simulink model "Simulink_Program"  (R2023b)
settings: Solver=VariableStepAuto  StartTime=0.0  StopTime=1  RelTol=1e-3
undefined symbols (not defined in the file): battery_builder_rtmsupport, gcbh, Ns_Module, NumModules
libraries: nesl_utility x52, BatteryPack_105s34p_Library_lib x36, fl_lib x17, ee_lib x7
(part 2 of 5)

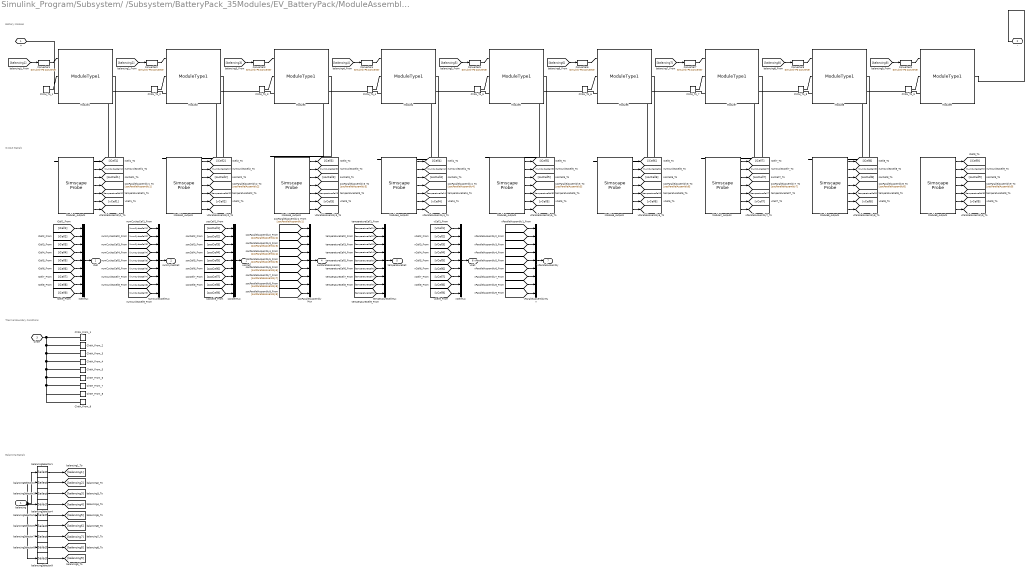
== system Simulink_Program/Subsystem/ /Subsystem/BatteryPack_35Modules/EV_BatteryPack/ModuleAssembly1 ==
  note: Balancing Signals
  note: Thermal Boundary Conditions
  note: Output Signals
  note: Battery Modules
  balancing : Inport  PortDimensions=27
  ClntH_From_1 : ConnectionLabel  Label=clntH_1
  ClntH_From_2 : ConnectionLabel  Label=clntH_2
  ClntH_From_3 : ConnectionLabel  Label=clntH_3
  ClntH_From_4 : ConnectionLabel  Label=clntH_4
  ClntH_From_5 : ConnectionLabel  Label=clntH_5
  ClntH_From_6 : ConnectionLabel  Label=clntH_6
  ClntH_From_7 : ConnectionLabel  Label=clntH_7
  ClntH_From_8 : ConnectionLabel  Label=clntH_8
  ClntH_From_9 : ConnectionLabel  Label=clntH_9
  ClntH_To_1 : ConnectionLabel  Label=clntH_1
  ClntH_To_2 : ConnectionLabel  Label=clntH_2
  ClntH_To_3 : ConnectionLabel  Label=clntH_3
  ClntH_To_4 : ConnectionLabel  Label=clntH_4
  ClntH_To_5 : ConnectionLabel  Label=clntH_5
  ClntH_To_6 : ConnectionLabel  Label=clntH_6
  ClntH_To_7 : ConnectionLabel  Label=clntH_7
  ClntH_To_8 : ConnectionLabel  Label=clntH_8
  ClntH_To_9 : ConnectionLabel  Label=clntH_9
  Converter{1..9} (9 alike) : nesl_utility/Simulink-PS Converter  PhysicalDomain=network_engine_domain  SubClassName=ps_input  LeftPortType=input  RightPortType=output  PseudoPeriodic=off  Frequencies=[]  NoiseDistribution=none  NoiseParameters=[]  Unit=1  AffineConversion=off  FilteringAndDerivatives=provide  SimscapeFilterOrder=1  InputFilterTimeConstant=0.001  UdotUserProvided=0
  Module1 : BatteryPack_105s34p_Library_lib/Modules/ModuleType1  SOC_vecCell=ModuleType1.SOC_vecCell  T_vecCell=ModuleType1.T_vecCell K  V0_matCell=ModuleType1.V0_matCell V  V_rangeCell=ModuleType1.V_rangeCell V  R0_matCell=ModuleType1.R0_matCell Ohm  AHCell=ModuleType1.AHCell A*hr  extrapolation_optionCell=simscape.enum.extrapolation.nearest  thermal_massCell=ModuleType1.thermal_massCell J/K  CoolantResistance=ModuleType1.CoolantResistance K/W  CellBalancingClosedResistance=ModuleType1.CellBalancingClosedResistance Ohm  CellBalancingOpenConductance=ModuleType1.CellBalancingOpenConductance 1/Ohm  CellBalancingThreshold=ModuleType1.CellBalancingThreshold  CellBalancingResistance=ModuleType1.CellBalancingResistance Ohm  P=34  S=3  iCell_specify=on  iCell_priority=None  iCell=ModuleAssembly1.Module1.iCell A  iCell_nominal_specify=off  iCell_nominal_unit=A  iCell_nominal_value=1  vCell_specify=on  vCell_priority=None  vCell=ModuleAssembly1.Module1.vCell V  vCell_nominal_specify=off  vCell_nominal_unit=V  vCell_nominal_value=1  socCell_specify=on  socCell_priority=High  socCell=ModuleAssembly1.Module1.socCell  socCell_nominal_specify=off  socCell_nominal_unit=1  socCell_nominal_value=1  numCyclesCell_specify=on  numCyclesCell_priority=High  numCyclesCell=ModuleAssembly1.Module1.numCyclesCell  numCyclesCell_nominal_specify=off  numCyclesCell_nominal_unit=1  numCyclesCell_nominal_value=1  temperatureCell_specify=on  temperatureCell_priority=High  temperatureCell=ModuleAssembly1.Module1.temperatureCell K  temperatureCell_nominal_specify=off  temperatureCell_nominal_unit=K  temperatureCell_nominal_value=1  vParallelAssembly_specify=on  vParallelAssembly_priority=None  vParallelAssembly=ModuleAssembly1.Module1.vParallelAssembly V  vParallelAssembly_nominal_specify=off  vParallelAssembly_nominal_unit=V  vParallelAssembly_nominal_value=1  socParallelAssembly_specify=on  socParallelAssembly_priority=None  socParallelAssembly=ModuleAssembly1.Module1.socParallelAssembly  socParallelAssembly_nominal_specify=off  socParallelAssembly_nominal_unit=1  socParallelAssembly_nominal_value=1
      settings: InternalSimscapePortConfiguration="{\"Bottom\":[{\"id\":\"n\",\"label\":\"-\",\"type\":\"foundation.electrical.electrical\"}],\"Left\":[{\"id\":\"enableCellBalancing\",\"label\":\"CB\",\"type\":\"input\"},{\"id\":\"ClntH\",\"label\":\"ClntH\",\"type\":\"foundation.thermal.thermal\"}],\"Right\":[],\"Top\":[{\"id\":\"p\",\"label\":\"+\",\"type\":\"foundation.electrical.electrical\"}]}"
  Module1_outputs : SimscapeProbe  BoundBlock=363  Variables={iCell, numCyclesCell, socCell, socParallelAssembly, temperatureCell, vCell, vParallelAssembly}
  Module2 : BatteryPack_105s34p_Library_lib/Modules/ModuleType1  SOC_vecCell=ModuleType1.SOC_vecCell  T_vecCell=ModuleType1.T_vecCell K  V0_matCell=ModuleType1.V0_matCell V  V_rangeCell=ModuleType1.V_rangeCell V  R0_matCell=ModuleType1.R0_matCell Ohm  AHCell=ModuleType1.AHCell A*hr  extrapolation_optionCell=simscape.enum.extrapolation.nearest  thermal_massCell=ModuleType1.thermal_massCell J/K  CoolantResistance=ModuleType1.CoolantResistance K/W  CellBalancingClosedResistance=ModuleType1.CellBalancingClosedResistance Ohm  CellBalancingOpenConductance=ModuleType1.CellBalancingOpenConductance 1/Ohm  CellBalancingThreshold=ModuleType1.CellBalancingThreshold  CellBalancingResistance=ModuleType1.CellBalancingResistance Ohm  P=34  S=3  iCell_specify=on  iCell_priority=None  iCell=ModuleAssembly1.Module2.iCell A  iCell_nominal_specify=off  iCell_nominal_unit=A  iCell_nominal_value=1  vCell_specify=on  vCell_priority=None  vCell=ModuleAssembly1.Module2.vCell V  vCell_nominal_specify=off  vCell_nominal_unit=V  vCell_nominal_value=1  socCell_specify=on  socCell_priority=High  socCell=ModuleAssembly1.Module2.socCell  socCell_nominal_specify=off  socCell_nominal_unit=1  socCell_nominal_value=1  numCyclesCell_specify=on  numCyclesCell_priority=High  numCyclesCell=ModuleAssembly1.Module2.numCyclesCell  numCyclesCell_nominal_specify=off  numCyclesCell_nominal_unit=1  numCyclesCell_nominal_value=1  temperatureCell_specify=on  temperatureCell_priority=High  temperatureCell=ModuleAssembly1.Module2.temperatureCell K  temperatureCell_nominal_specify=off  temperatureCell_nominal_unit=K  temperatureCell_nominal_value=1  vParallelAssembly_specify=on  vParallelAssembly_priority=None  vParallelAssembly=ModuleAssembly1.Module2.vParallelAssembly V  vParallelAssembly_nominal_specify=off  vParallelAssembly_nominal_unit=V  vParallelAssembly_nominal_value=1  socParallelAssembly_specify=on  socParallelAssembly_priority=None  socParallelAssembly=ModuleAssembly1.Module2.socParallelAssembly  socParallelAssembly_nominal_specify=off  socParallelAssembly_nominal_unit=1  socParallelAssembly_nominal_value=1
      settings: InternalSimscapePortConfiguration="{\"Bottom\":[{\"id\":\"n\",\"label\":\"-\",\"type\":\"foundation.electrical.electrical\"}],\"Left\":[{\"id\":\"enableCellBalancing\",\"label\":\"CB\",\"type\":\"input\"},{\"id\":\"ClntH\",\"label\":\"ClntH\",\"type\":\"foundation.thermal.thermal\"}],\"Right\":[],\"Top\":[{\"id\":\"p\",\"label\":\"+\",\"type\":\"foundation.electrical.electrical\"}]}"
  Module2_outputs : SimscapeProbe  BoundBlock=365  Variables={iCell, numCyclesCell, socCell, socParallelAssembly, temperatureCell, vCell, vParallelAssembly}
  Module3 : BatteryPack_105s34p_Library_lib/Modules/ModuleType1  SOC_vecCell=ModuleType1.SOC_vecCell  T_vecCell=ModuleType1.T_vecCell K  V0_matCell=ModuleType1.V0_matCell V  V_rangeCell=ModuleType1.V_rangeCell V  R0_matCell=ModuleType1.R0_matCell Ohm  AHCell=ModuleType1.AHCell A*hr  extrapolation_optionCell=simscape.enum.extrapolation.nearest  thermal_massCell=ModuleType1.thermal_massCell J/K  CoolantResistance=ModuleType1.CoolantResistance K/W  CellBalancingClosedResistance=ModuleType1.CellBalancingClosedResistance Ohm  CellBalancingOpenConductance=ModuleType1.CellBalancingOpenConductance 1/Ohm  CellBalancingThreshold=ModuleType1.CellBalancingThreshold  CellBalancingResistance=ModuleType1.CellBalancingResistance Ohm  P=34  S=3  iCell_specify=on  iCell_priority=None  iCell=ModuleAssembly1.Module3.iCell A  iCell_nominal_specify=off  iCell_nominal_unit=A  iCell_nominal_value=1  vCell_specify=on  vCell_priority=None  vCell=ModuleAssembly1.Module3.vCell V  vCell_nominal_specify=off  vCell_nominal_unit=V  vCell_nominal_value=1  socCell_specify=on  socCell_priority=High  socCell=ModuleAssembly1.Module3.socCell  socCell_nominal_specify=off  socCell_nominal_unit=1  socCell_nominal_value=1  numCyclesCell_specify=on  numCyclesCell_priority=High  numCyclesCell=ModuleAssembly1.Module3.numCyclesCell  numCyclesCell_nominal_specify=off  numCyclesCell_nominal_unit=1  numCyclesCell_nominal_value=1  temperatureCell_specify=on  temperatureCell_priority=High  temperatureCell=ModuleAssembly1.Module3.temperatureCell K  temperatureCell_nominal_specify=off  temperatureCell_nominal_unit=K  temperatureCell_nominal_value=1  vParallelAssembly_specify=on  vParallelAssembly_priority=None  vParallelAssembly=ModuleAssembly1.Module3.vParallelAssembly V  vParallelAssembly_nominal_specify=off  vParallelAssembly_nominal_unit=V  vParallelAssembly_nominal_value=1  socParallelAssembly_specify=on  socParallelAssembly_priority=None  socParallelAssembly=ModuleAssembly1.Module3.socParallelAssembly  socParallelAssembly_nominal_specify=off  socParallelAssembly_nominal_unit=1  socParallelAssembly_nominal_value=1
      settings: InternalSimscapePortConfiguration="{\"Bottom\":[{\"id\":\"n\",\"label\":\"-\",\"type\":\"foundation.electrical.electrical\"}],\"Left\":[{\"id\":\"enableCellBalancing\",\"label\":\"CB\",\"type\":\"input\"},{\"id\":\"ClntH\",\"label\":\"ClntH\",\"type\":\"foundation.thermal.thermal\"}],\"Right\":[],\"Top\":[{\"id\":\"p\",\"label\":\"+\",\"type\":\"foundation.electrical.electrical\"}]}"
  Module3_outputs : SimscapeProbe  BoundBlock=367  Variables={iCell, numCyclesCell, socCell, socParallelAssembly, temperatureCell, vCell, vParallelAssembly}
  Module4 : BatteryPack_105s34p_Library_lib/Modules/ModuleType1  SOC_vecCell=ModuleType1.SOC_vecCell  T_vecCell=ModuleType1.T_vecCell K  V0_matCell=ModuleType1.V0_matCell V  V_rangeCell=ModuleType1.V_rangeCell V  R0_matCell=ModuleType1.R0_matCell Ohm  AHCell=ModuleType1.AHCell A*hr  extrapolation_optionCell=simscape.enum.extrapolation.nearest  thermal_massCell=ModuleType1.thermal_massCell J/K  CoolantResistance=ModuleType1.CoolantResistance K/W  CellBalancingClosedResistance=ModuleType1.CellBalancingClosedResistance Ohm  CellBalancingOpenConductance=ModuleType1.CellBalancingOpenConductance 1/Ohm  CellBalancingThreshold=ModuleType1.CellBalancingThreshold  CellBalancingResistance=ModuleType1.CellBalancingResistance Ohm  P=34  S=3  iCell_specify=on  iCell_priority=None  iCell=ModuleAssembly1.Module4.iCell A  iCell_nominal_specify=off  iCell_nominal_unit=A  iCell_nominal_value=1  vCell_specify=on  vCell_priority=None  vCell=ModuleAssembly1.Module4.vCell V  vCell_nominal_specify=off  vCell_nominal_unit=V  vCell_nominal_value=1  socCell_specify=on  socCell_priority=High  socCell=ModuleAssembly1.Module4.socCell  socCell_nominal_specify=off  socCell_nominal_unit=1  socCell_nominal_value=1  numCyclesCell_specify=on  numCyclesCell_priority=High  numCyclesCell=ModuleAssembly1.Module4.numCyclesCell  numCyclesCell_nominal_specify=off  numCyclesCell_nominal_unit=1  numCyclesCell_nominal_value=1  temperatureCell_specify=on  temperatureCell_priority=High  temperatureCell=ModuleAssembly1.Module4.temperatureCell K  temperatureCell_nominal_specify=off  temperatureCell_nominal_unit=K  temperatureCell_nominal_value=1  vParallelAssembly_specify=on  vParallelAssembly_priority=None  vParallelAssembly=ModuleAssembly1.Module4.vParallelAssembly V  vParallelAssembly_nominal_specify=off  vParallelAssembly_nominal_unit=V  vParallelAssembly_nominal_value=1  socParallelAssembly_specify=on  socParallelAssembly_priority=None  socParallelAssembly=ModuleAssembly1.Module4.socParallelAssembly  socParallelAssembly_nominal_specify=off  socParallelAssembly_nominal_unit=1  socParallelAssembly_nominal_value=1
      settings: InternalSimscapePortConfiguration="{\"Bottom\":[{\"id\":\"n\",\"label\":\"-\",\"type\":\"foundation.electrical.electrical\"}],\"Left\":[{\"id\":\"enableCellBalancing\",\"label\":\"CB\",\"type\":\"input\"},{\"id\":\"ClntH\",\"label\":\"ClntH\",\"type\":\"foundation.thermal.thermal\"}],\"Right\":[],\"Top\":[{\"id\":\"p\",\"label\":\"+\",\"type\":\"foundation.electrical.electrical\"}]}"
  Module4_outputs : SimscapeProbe  BoundBlock=369  Variables={iCell, numCyclesCell, socCell, socParallelAssembly, temperatureCell, vCell, vParallelAssembly}
  Module5 : BatteryPack_105s34p_Library_lib/Modules/ModuleType1  SOC_vecCell=ModuleType1.SOC_vecCell  T_vecCell=ModuleType1.T_vecCell K  V0_matCell=ModuleType1.V0_matCell V  V_rangeCell=ModuleType1.V_rangeCell V  R0_matCell=ModuleType1.R0_matCell Ohm  AHCell=ModuleType1.AHCell A*hr  extrapolation_optionCell=simscape.enum.extrapolation.nearest  thermal_massCell=ModuleType1.thermal_massCell J/K  CoolantResistance=ModuleType1.CoolantResistance K/W  CellBalancingClosedResistance=ModuleType1.CellBalancingClosedResistance Ohm  CellBalancingOpenConductance=ModuleType1.CellBalancingOpenConductance 1/Ohm  CellBalancingThreshold=ModuleType1.CellBalancingThreshold  CellBalancingResistance=ModuleType1.CellBalancingResistance Ohm  P=34  S=3  iCell_specify=on  iCell_priority=None  iCell=ModuleAssembly1.Module5.iCell A  iCell_nominal_specify=off  iCell_nominal_unit=A  iCell_nominal_value=1  vCell_specify=on  vCell_priority=None  vCell=ModuleAssembly1.Module5.vCell V  vCell_nominal_specify=off  vCell_nominal_unit=V  vCell_nominal_value=1  socCell_specify=on  socCell_priority=High  socCell=ModuleAssembly1.Module5.socCell  socCell_nominal_specify=off  socCell_nominal_unit=1  socCell_nominal_value=1  numCyclesCell_specify=on  numCyclesCell_priority=High  numCyclesCell=ModuleAssembly1.Module5.numCyclesCell  numCyclesCell_nominal_specify=off  numCyclesCell_nominal_unit=1  numCyclesCell_nominal_value=1  temperatureCell_specify=on  temperatureCell_priority=High  temperatureCell=ModuleAssembly1.Module5.temperatureCell K  temperatureCell_nominal_specify=off  temperatureCell_nominal_unit=K  temperatureCell_nominal_value=1  vParallelAssembly_specify=on  vParallelAssembly_priority=None  vParallelAssembly=ModuleAssembly1.Module5.vParallelAssembly V  vParallelAssembly_nominal_specify=off  vParallelAssembly_nominal_unit=V  vParallelAssembly_nominal_value=1  socParallelAssembly_specify=on  socParallelAssembly_priority=None  socParallelAssembly=ModuleAssembly1.Module5.socParallelAssembly  socParallelAssembly_nominal_specify=off  socParallelAssembly_nominal_unit=1  socParallelAssembly_nominal_value=1
      settings: InternalSimscapePortConfiguration="{\"Bottom\":[{\"id\":\"n\",\"label\":\"-\",\"type\":\"foundation.electrical.electrical\"}],\"Left\":[{\"id\":\"enableCellBalancing\",\"label\":\"CB\",\"type\":\"input\"},{\"id\":\"ClntH\",\"label\":\"ClntH\",\"type\":\"foundation.thermal.thermal\"}],\"Right\":[],\"Top\":[{\"id\":\"p\",\"label\":\"+\",\"type\":\"foundation.electrical.electrical\"}]}"
  Module5_outputs : SimscapeProbe  BoundBlock=371  Variables={iCell, numCyclesCell, socCell, socParallelAssembly, temperatureCell, vCell, vParallelAssembly}
  Module6 : BatteryPack_105s34p_Library_lib/Modules/ModuleType1  SOC_vecCell=ModuleType1.SOC_vecCell  T_vecCell=ModuleType1.T_vecCell K  V0_matCell=ModuleType1.V0_matCell V  V_rangeCell=ModuleType1.V_rangeCell V  R0_matCell=ModuleType1.R0_matCell Ohm  AHCell=ModuleType1.AHCell A*hr  extrapolation_optionCell=simscape.enum.extrapolation.nearest  thermal_massCell=ModuleType1.thermal_massCell J/K  CoolantResistance=ModuleType1.CoolantResistance K/W  CellBalancingClosedResistance=ModuleType1.CellBalancingClosedResistance Ohm  CellBalancingOpenConductance=ModuleType1.CellBalancingOpenConductance 1/Ohm  CellBalancingThreshold=ModuleType1.CellBalancingThreshold  CellBalancingResistance=ModuleType1.CellBalancingResistance Ohm  P=34  S=3  iCell_specify=on  iCell_priority=None  iCell=ModuleAssembly1.Module6.iCell A  iCell_nominal_specify=off  iCell_nominal_unit=A  iCell_nominal_value=1  vCell_specify=on  vCell_priority=None  vCell=ModuleAssembly1.Module6.vCell V  vCell_nominal_specify=off  vCell_nominal_unit=V  vCell_nominal_value=1  socCell_specify=on  socCell_priority=High  socCell=ModuleAssembly1.Module6.socCell  socCell_nominal_specify=off  socCell_nominal_unit=1  socCell_nominal_value=1  numCyclesCell_specify=on  numCyclesCell_priority=High  numCyclesCell=ModuleAssembly1.Module6.numCyclesCell  numCyclesCell_nominal_specify=off  numCyclesCell_nominal_unit=1  numCyclesCell_nominal_value=1  temperatureCell_specify=on  temperatureCell_priority=High  temperatureCell=ModuleAssembly1.Module6.temperatureCell K  temperatureCell_nominal_specify=off  temperatureCell_nominal_unit=K  temperatureCell_nominal_value=1  vParallelAssembly_specify=on  vParallelAssembly_priority=None  vParallelAssembly=ModuleAssembly1.Module6.vParallelAssembly V  vParallelAssembly_nominal_specify=off  vParallelAssembly_nominal_unit=V  vParallelAssembly_nominal_value=1  socParallelAssembly_specify=on  socParallelAssembly_priority=None  socParallelAssembly=ModuleAssembly1.Module6.socParallelAssembly  socParallelAssembly_nominal_specify=off  socParallelAssembly_nominal_unit=1  socParallelAssembly_nominal_value=1
      settings: InternalSimscapePortConfiguration="{\"Bottom\":[{\"id\":\"n\",\"label\":\"-\",\"type\":\"foundation.electrical.electrical\"}],\"Left\":[{\"id\":\"enableCellBalancing\",\"label\":\"CB\",\"type\":\"input\"},{\"id\":\"ClntH\",\"label\":\"ClntH\",\"type\":\"foundation.thermal.thermal\"}],\"Right\":[],\"Top\":[{\"id\":\"p\",\"label\":\"+\",\"type\":\"foundation.electrical.electrical\"}]}"
  Module6_outputs : SimscapeProbe  BoundBlock=373  Variables={iCell, numCyclesCell, socCell, socParallelAssembly, temperatureCell, vCell, vParallelAssembly}
  Module7 : BatteryPack_105s34p_Library_lib/Modules/ModuleType1  SOC_vecCell=ModuleType1.SOC_vecCell  T_vecCell=ModuleType1.T_vecCell K  V0_matCell=ModuleType1.V0_matCell V  V_rangeCell=ModuleType1.V_rangeCell V  R0_matCell=ModuleType1.R0_matCell Ohm  AHCell=ModuleType1.AHCell A*hr  extrapolation_optionCell=simscape.enum.extrapolation.nearest  thermal_massCell=ModuleType1.thermal_massCell J/K  CoolantResistance=ModuleType1.CoolantResistance K/W  CellBalancingClosedResistance=ModuleType1.CellBalancingClosedResistance Ohm  CellBalancingOpenConductance=ModuleType1.CellBalancingOpenConductance 1/Ohm  CellBalancingThreshold=ModuleType1.CellBalancingThreshold  CellBalancingResistance=ModuleType1.CellBalancingResistance Ohm  P=34  S=3  iCell_specify=on  iCell_priority=None  iCell=ModuleAssembly1.Module7.iCell A  iCell_nominal_specify=off  iCell_nominal_unit=A  iCell_nominal_value=1  vCell_specify=on  vCell_priority=None  vCell=ModuleAssembly1.Module7.vCell V  vCell_nominal_specify=off  vCell_nominal_unit=V  vCell_nominal_value=1  socCell_specify=on  socCell_priority=High  socCell=ModuleAssembly1.Module7.socCell  socCell_nominal_specify=off  socCell_nominal_unit=1  socCell_nominal_value=1  numCyclesCell_specify=on  numCyclesCell_priority=High  numCyclesCell=ModuleAssembly1.Module7.numCyclesCell  numCyclesCell_nominal_specify=off  numCyclesCell_nominal_unit=1  numCyclesCell_nominal_value=1  temperatureCell_specify=on  temperatureCell_priority=High  temperatureCell=ModuleAssembly1.Module7.temperatureCell K  temperatureCell_nominal_specify=off  temperatureCell_nominal_unit=K  temperatureCell_nominal_value=1  vParallelAssembly_specify=on  vParallelAssembly_priority=None  vParallelAssembly=ModuleAssembly1.Module7.vParallelAssembly V  vParallelAssembly_nominal_specify=off  vParallelAssembly_nominal_unit=V  vParallelAssembly_nominal_value=1  socParallelAssembly_specify=on  socParallelAssembly_priority=None  socParallelAssembly=ModuleAssembly1.Module7.socParallelAssembly  socParallelAssembly_nominal_specify=off  socParallelAssembly_nominal_unit=1  socParallelAssembly_nominal_value=1
      settings: InternalSimscapePortConfiguration="{\"Bottom\":[{\"id\":\"n\",\"label\":\"-\",\"type\":\"foundation.electrical.electrical\"}],\"Left\":[{\"id\":\"enableCellBalancing\",\"label\":\"CB\",\"type\":\"input\"},{\"id\":\"ClntH\",\"label\":\"ClntH\",\"type\":\"foundation.thermal.thermal\"}],\"Right\":[],\"Top\":[{\"id\":\"p\",\"label\":\"+\",\"type\":\"foundation.electrical.electrical\"}]}"
  Module7_outputs : SimscapeProbe  BoundBlock=375  Variables={iCell, numCyclesCell, socCell, socParallelAssembly, temperatureCell, vCell, vParallelAssembly}
  Module8 : BatteryPack_105s34p_Library_lib/Modules/ModuleType1  SOC_vecCell=ModuleType1.SOC_vecCell  T_vecCell=ModuleType1.T_vecCell K  V0_matCell=ModuleType1.V0_matCell V  V_rangeCell=ModuleType1.V_rangeCell V  R0_matCell=ModuleType1.R0_matCell Ohm  AHCell=ModuleType1.AHCell A*hr  extrapolation_optionCell=simscape.enum.extrapolation.nearest  thermal_massCell=ModuleType1.thermal_massCell J/K  CoolantResistance=ModuleType1.CoolantResistance K/W  CellBalancingClosedResistance=ModuleType1.CellBalancingClosedResistance Ohm  CellBalancingOpenConductance=ModuleType1.CellBalancingOpenConductance 1/Ohm  CellBalancingThreshold=ModuleType1.CellBalancingThreshold  CellBalancingResistance=ModuleType1.CellBalancingResistance Ohm  P=34  S=3  iCell_specify=on  iCell_priority=None  iCell=ModuleAssembly1.Module8.iCell A  iCell_nominal_specify=off  iCell_nominal_unit=A  iCell_nominal_value=1  vCell_specify=on  vCell_priority=None  vCell=ModuleAssembly1.Module8.vCell V  vCell_nominal_specify=off  vCell_nominal_unit=V  vCell_nominal_value=1  socCell_specify=on  socCell_priority=High  socCell=ModuleAssembly1.Module8.socCell  socCell_nominal_specify=off  socCell_nominal_unit=1  socCell_nominal_value=1  numCyclesCell_specify=on  numCyclesCell_priority=High  numCyclesCell=ModuleAssembly1.Module8.numCyclesCell  numCyclesCell_nominal_specify=off  numCyclesCell_nominal_unit=1  numCyclesCell_nominal_value=1  temperatureCell_specify=on  temperatureCell_priority=High  temperatureCell=ModuleAssembly1.Module8.temperatureCell K  temperatureCell_nominal_specify=off  temperatureCell_nominal_unit=K  temperatureCell_nominal_value=1  vParallelAssembly_specify=on  vParallelAssembly_priority=None  vParallelAssembly=ModuleAssembly1.Module8.vParallelAssembly V  vParallelAssembly_nominal_specify=off  vParallelAssembly_nominal_unit=V  vParallelAssembly_nominal_value=1  socParallelAssembly_specify=on  socParallelAssembly_priority=None  socParallelAssembly=ModuleAssembly1.Module8.socParallelAssembly  socParallelAssembly_nominal_specify=off  socParallelAssembly_nominal_unit=1  socParallelAssembly_nominal_value=1
      settings: InternalSimscapePortConfiguration="{\"Bottom\":[{\"id\":\"n\",\"label\":\"-\",\"type\":\"foundation.electrical.electrical\"}],\"Left\":[{\"id\":\"enableCellBalancing\",\"label\":\"CB\",\"type\":\"input\"},{\"id\":\"ClntH\",\"label\":\"ClntH\",\"type\":\"foundation.thermal.thermal\"}],\"Right\":[],\"Top\":[{\"id\":\"p\",\"label\":\"+\",\"type\":\"foundation.electrical.electrical\"}]}"
  Module8_outputs : SimscapeProbe  BoundBlock=377  Variables={iCell, numCyclesCell, socCell, socParallelAssembly, temperatureCell, vCell, vParallelAssembly}
  Module9 : BatteryPack_105s34p_Library_lib/Modules/ModuleType1  SOC_vecCell=ModuleType1.SOC_vecCell  T_vecCell=ModuleType1.T_vecCell K  V0_matCell=ModuleType1.V0_matCell V  V_rangeCell=ModuleType1.V_rangeCell V  R0_matCell=ModuleType1.R0_matCell Ohm  AHCell=ModuleType1.AHCell A*hr  extrapolation_optionCell=simscape.enum.extrapolation.nearest  thermal_massCell=ModuleType1.thermal_massCell J/K  CoolantResistance=ModuleType1.CoolantResistance K/W  CellBalancingClosedResistance=ModuleType1.CellBalancingClosedResistance Ohm  CellBalancingOpenConductance=ModuleType1.CellBalancingOpenConductance 1/Ohm  CellBalancingThreshold=ModuleType1.CellBalancingThreshold  CellBalancingResistance=ModuleType1.CellBalancingResistance Ohm  P=34  S=3  iCell_specify=on  iCell_priority=None  iCell=ModuleAssembly1.Module9.iCell A  iCell_nominal_specify=off  iCell_nominal_unit=A  iCell_nominal_value=1  vCell_specify=on  vCell_priority=None  vCell=ModuleAssembly1.Module9.vCell V  vCell_nominal_specify=off  vCell_nominal_unit=V  vCell_nominal_value=1  socCell_specify=on  socCell_priority=High  socCell=ModuleAssembly1.Module9.socCell  socCell_nominal_specify=off  socCell_nominal_unit=1  socCell_nominal_value=1  numCyclesCell_specify=on  numCyclesCell_priority=High  numCyclesCell=ModuleAssembly1.Module9.numCyclesCell  numCyclesCell_nominal_specify=off  numCyclesCell_nominal_unit=1  numCyclesCell_nominal_value=1  temperatureCell_specify=on  temperatureCell_priority=High  temperatureCell=ModuleAssembly1.Module9.temperatureCell K  temperatureCell_nominal_specify=off  temperatureCell_nominal_unit=K  temperatureCell_nominal_value=1  vParallelAssembly_specify=on  vParallelAssembly_priority=None  vParallelAssembly=ModuleAssembly1.Module9.vParallelAssembly V  vParallelAssembly_nominal_specify=off  vParallelAssembly_nominal_unit=V  vParallelAssembly_nominal_value=1  socParallelAssembly_specify=on  socParallelAssembly_priority=None  socParallelAssembly=ModuleAssembly1.Module9.socParallelAssembly  socParallelAssembly_nominal_specify=off  socParallelAssembly_nominal_unit=1  socParallelAssembly_nominal_value=1
      settings: InternalSimscapePortConfiguration="{\"Bottom\":[{\"id\":\"n\",\"label\":\"-\",\"type\":\"foundation.electrical.electrical\"}],\"Left\":[{\"id\":\"enableCellBalancing\",\"label\":\"CB\",\"type\":\"input\"},{\"id\":\"ClntH\",\"label\":\"ClntH\",\"type\":\"foundation.thermal.thermal\"}],\"Right\":[],\"Top\":[{\"id\":\"p\",\"label\":\"+\",\"type\":\"foundation.electrical.electrical\"}]}"
  Module9_outputs : SimscapeProbe  BoundBlock=379  Variables={iCell, numCyclesCell, socCell, socParallelAssembly, temperatureCell, vCell, vParallelAssembly}
  balancingSelector1 : Selector  InputPortWidth=27  IndexOptions=Index vector (dialog)  Indices="[1  2  3]"  OutputSizes=1
  balancingSelector2 : Selector  InputPortWidth=27  IndexOptions=Index vector (dialog)  Indices="[4  5  6]"  OutputSizes=1
  balancingSelector3 : Selector  InputPortWidth=27  IndexOptions=Index vector (dialog)  Indices="[7  8  9]"  OutputSizes=1
  balancingSelector4 : Selector  InputPortWidth=27  IndexOptions=Index vector (dialog)  Indices="[10  11  12]"  OutputSizes=1
  balancingSelector5 : Selector  InputPortWidth=27  IndexOptions=Index vector (dialog)  Indices="[13  14  15]"  OutputSizes=1
  balancingSelector6 : Selector  InputPortWidth=27  IndexOptions=Index vector (dialog)  Indices="[16  17  18]"  OutputSizes=1
  balancingSelector7 : Selector  InputPortWidth=27  IndexOptions=Index vector (dialog)  Indices="[19  20  21]"  OutputSizes=1
  balancingSelector8 : Selector  InputPortWidth=27  IndexOptions=Index vector (dialog)  Indices="[22  23  24]"  OutputSizes=1
  balancingSelector9 : Selector  InputPortWidth=27  IndexOptions=Index vector (dialog)  Indices="[25  26  27]"  OutputSizes=1
  iCellMux : Mux  Inputs=9
  numCyclesCellMux : Mux  Inputs=9
  socCellMux : Mux  Inputs=9
  socParallelAssemblyMux : Mux  Inputs=9
  temperatureCellMux : Mux  Inputs=9
  vCellMux : Mux  Inputs=9
  vParallelAssemblyMux : Mux  Inputs=9
  + : PMIOPort  Side=Left
  - : PMIOPort  Port=2  Side=Right
  ClntH : PMIOPort  Port=3  Side=Right  ConnectionType=Connection: foundation.thermal.thermal
  iCell : Outport
  numCyclesCell : Outport  Port=2
  socCell : Outport  Port=3
  socParallelAssembly : Outport  Port=4
  temperatureCell : Outport  Port=5
  vCell : Outport  Port=6
  vParallelAssembly : Outport  Port=7
  wires:
  balancingSelector9/1 -> [balancing9]
  [balancing9] -> Converter9/1
  balancingSelector8/1 -> [balancing8]
  [balancing8] -> Converter8/1
  balancingSelector7/1 -> [balancing7]
  [balancing7] -> Converter7/1
  balancingSelector6/1 -> [balancing6]
  [balancing6] -> Converter6/1
  balancingSelector5/1 -> [balancing5]
  [balancing5] -> Converter5/1
  balancingSelector4/1 -> [balancing4]
  [balancing4] -> Converter4/1
  balancingSelector3/1 -> [balancing3]
  [balancing3] -> Converter3/1
  balancingSelector2/1 -> [balancing2]
  [balancing2] -> Converter2/1
  balancingSelector1/1 -> [balancing1]
  balancing/1 -> balancingSelector9/1, balancingSelector8/1, balancingSelector7/1, balancingSelector6/1, balancingSelector5/1, balancingSelector4/1, balancingSelector3/1, balancingSelector2/1, balancingSelector1/1
  [balancing1] -> Converter1/1
  [vParallelAssembly9] -> vParallelAssemblyMux/9
  Module9_outputs/7 -> [vParallelAssembly9]
  [vCell9] -> vCellMux/9
  Module9_outputs/6 -> [vCell9]
  [temperatureCell9] -> temperatureCellMux/9
  Module9_outputs/5 -> [temperatureCell9]
  [socParallelAssembly9] -> socParallelAssemblyMux/9
  Module9_outputs/4 -> [socParallelAssembly9]
  [socCell9] -> socCellMux/9
  Module9_outputs/3 -> [socCell9]
  [numCyclesCell9] -> numCyclesCellMux/9
  Module9_outputs/2 -> [numCyclesCell9]
  [iCell9] -> iCellMux/9
  Module9_outputs/1 -> [iCell9]
  [vParallelAssembly8] -> vParallelAssemblyMux/8
  Module8_outputs/7 -> [vParallelAssembly8]
  [vCell8] -> vCellMux/8
  Module8_outputs/6 -> [vCell8]
  [temperatureCell8] -> temperatureCellMux/8
  Module8_outputs/5 -> [temperatureCell8]
  [socParallelAssembly8] -> socParallelAssemblyMux/8
  Module8_outputs/4 -> [socParallelAssembly8]
  [socCell8] -> socCellMux/8
  Module8_outputs/3 -> [socCell8]
  [numCyclesCell8] -> numCyclesCellMux/8
  Module8_outputs/2 -> [numCyclesCell8]
  [iCell8] -> iCellMux/8
  Module8_outputs/1 -> [iCell8]
  [vParallelAssembly7] -> vParallelAssemblyMux/7
  Module7_outputs/7 -> [vParallelAssembly7]
  [vCell7] -> vCellMux/7
  Module7_outputs/6 -> [vCell7]
  [temperatureCell7] -> temperatureCellMux/7
  Module7_outputs/5 -> [temperatureCell7]
  [socParallelAssembly7] -> socParallelAssemblyMux/7
  Module7_outputs/4 -> [socParallelAssembly7]
  [socCell7] -> socCellMux/7
  Module7_outputs/3 -> [socCell7]
  [numCyclesCell7] -> numCyclesCellMux/7
  Module7_outputs/2 -> [numCyclesCell7]
  [iCell7] -> iCellMux/7
  Module7_outputs/1 -> [iCell7]
  [vParallelAssembly6] -> vParallelAssemblyMux/6
  Module6_outputs/7 -> [vParallelAssembly6]
  [vCell6] -> vCellMux/6
  Module6_outputs/6 -> [vCell6]
  [temperatureCell6] -> temperatureCellMux/6
  Module6_outputs/5 -> [temperatureCell6]
  [socParallelAssembly6] -> socParallelAssemblyMux/6
  Module6_outputs/4 -> [socParallelAssembly6]
  [socCell6] -> socCellMux/6
  Module6_outputs/3 -> [socCell6]
  [numCyclesCell6] -> numCyclesCellMux/6
  Module6_outputs/2 -> [numCyclesCell6]
  [iCell6] -> iCellMux/6
  Module6_outputs/1 -> [iCell6]
  [vParallelAssembly5] -> vParallelAssemblyMux/5
  Module5_outputs/7 -> [vParallelAssembly5]
  [vCell5] -> vCellMux/5
  Module5_outputs/6 -> [vCell5]
  [temperatureCell5] -> temperatureCellMux/5
  Module5_outputs/5 -> [temperatureCell5]
  [socParallelAssembly5] -> socParallelAssemblyMux/5
  Module5_outputs/4 -> [socParallelAssembly5]
  [socCell5] -> socCellMux/5
  Module5_outputs/3 -> [socCell5]
  [numCyclesCell5] -> numCyclesCellMux/5
  Module5_outputs/2 -> [numCyclesCell5]
  [iCell5] -> iCellMux/5
  Module5_outputs/1 -> [iCell5]
  [vParallelAssembly4] -> vParallelAssemblyMux/4
  Module4_outputs/7 -> [vParallelAssembly4]
  [vCell4] -> vCellMux/4
  Module4_outputs/6 -> [vCell4]
  [temperatureCell4] -> temperatureCellMux/4
  Module4_outputs/5 -> [temperatureCell4]
  [socParallelAssembly4] -> socParallelAssemblyMux/4
  Module4_outputs/4 -> [socParallelAssembly4]
  [socCell4] -> socCellMux/4
  Module4_outputs/3 -> [socCell4]
  [numCyclesCell4] -> numCyclesCellMux/4
  Module4_outputs/2 -> [numCyclesCell4]
  [iCell4] -> iCellMux/4
  Module4_outputs/1 -> [iCell4]
  [vParallelAssembly3] -> vParallelAssemblyMux/3
  Module3_outputs/7 -> [vParallelAssembly3]
  [vCell3] -> vCellMux/3
  Module3_outputs/6 -> [vCell3]
  [temperatureCell3] -> temperatureCellMux/3
  Module3_outputs/5 -> [temperatureCell3]
  [socParallelAssembly3] -> socParallelAssemblyMux/3
  Module3_outputs/4 -> [socParallelAssembly3]
  [socCell3] -> socCellMux/3
  Module3_outputs/3 -> [socCell3]
  [numCyclesCell3] -> numCyclesCellMux/3
  Module3_outputs/2 -> [numCyclesCell3]
  [iCell3] -> iCellMux/3
  Module3_outputs/1 -> [iCell3]
  [vParallelAssembly2] -> vParallelAssemblyMux/2
  Module2_outputs/7 -> [vParallelAssembly2]
  [vCell2] -> vCellMux/2
  Module2_outputs/6 -> [vCell2]
  [temperatureCell2] -> temperatureCellMux/2
  Module2_outputs/5 -> [temperatureCell2]
  [socParallelAssembly2] -> socParallelAssemblyMux/2
  Module2_outputs/4 -> [socParallelAssembly2]
  [socCell2] -> socCellMux/2
  Module2_outputs/3 -> [socCell2]
  [numCyclesCell2] -> numCyclesCellMux/2
  Module2_outputs/2 -> [numCyclesCell2]
  [iCell2] -> iCellMux/2
  Module2_outputs/1 -> [iCell2]
  [vParallelAssembly1] -> vParallelAssemblyMux/1
  vParallelAssemblyMux/1 -> vParallelAssembly/1
  Module1_outputs/7 -> [vParallelAssembly1]
  [vCell1] -> vCellMux/1
  vCellMux/1 -> vCell/1
  Module1_outputs/6 -> [vCell1]
  [temperatureCell1] -> temperatureCellMux/1
  temperatureCellMux/1 -> temperatureCell/1
  Module1_outputs/5 -> [temperatureCell1]
  [socParallelAssembly1] -> socParallelAssemblyMux/1
  socParallelAssemblyMux/1 -> socParallelAssembly/1
  Module1_outputs/4 -> [socParallelAssembly1]
  [socCell1] -> socCellMux/1
  socCellMux/1 -> socCell/1
  Module1_outputs/3 -> [socCell1]
  [numCyclesCell1] -> numCyclesCellMux/1
  numCyclesCellMux/1 -> numCyclesCell/1
  Module1_outputs/2 -> [numCyclesCell1]
  [iCell1] -> iCellMux/1
  iCellMux/1 -> iCell/1
  Module1_outputs/1 -> [iCell1]
  connections:
  Converter9/RConn1 -- Module9/LConn1
  Converter8/RConn1 -- Module8/LConn1
  Converter7/RConn1 -- Module7/LConn1
  Converter6/RConn1 -- Module6/LConn1
  Converter5/RConn1 -- Module5/LConn1
  Converter4/RConn1 -- Module4/LConn1
  Converter3/RConn1 -- Module3/LConn1
  Converter2/RConn1 -- Module2/LConn1
  Converter1/RConn1 -- Module1/LConn1
  ClntH_To_9/LConn1 -- Module9/LConn2
  ClntH_To_8/LConn1 -- Module8/LConn2
  ClntH_To_7/LConn1 -- Module7/LConn2
  ClntH_To_6/LConn1 -- Module6/LConn2
  ClntH_To_5/LConn1 -- Module5/LConn2
  ClntH_To_4/LConn1 -- Module4/LConn2
  ClntH_To_3/LConn1 -- Module3/LConn2
  ClntH_To_2/LConn1 -- Module2/LConn2
  ClntH/RConn1 -- ClntH_From_1/LConn1 -- ClntH_From_2/LConn1 -- ClntH_From_3/LConn1 -- ClntH_From_4/LConn1 -- ClntH_From_5/LConn1 -- ClntH_From_6/LConn1 -- ClntH_From_7/LConn1 -- ClntH_From_9/LConn1 -- ClntH_From_8/LConn1
  ClntH_To_1/LConn1 -- Module1/LConn2
  Module9/RConn1 -- -/RConn1
  Module1/LConn3 -- +/RConn1
  Module9/LConn3 -- Module8/RConn1
  Module8/LConn3 -- Module7/RConn1
  Module7/LConn3 -- Module6/RConn1
  Module6/LConn3 -- Module5/RConn1
  Module5/LConn3 -- Module4/RConn1
  Module4/LConn3 -- Module3/RConn1
  Module3/LConn3 -- Module2/RConn1
  Module2/LConn3 -- Module1/RConn1
